simulink model "batteryModelFinal2019a"  (R2019a)
settings: Solver=VariableStepAuto  StartTime=0.0  StopTime=650  RelTol=1e-3
InitFcn:
  | load('batteryModelNew.mat');
  | load('soc_ocv_new.mat');
  | load('currentUAV.mat');
  | 
  | 
  | Q      = battery.QParam; % total capacity in mAh
  | n       = battery.etaParam; % coulombic efficiency
  | M      = battery.MParam; % dynamic hysteresis volts factor
  | Mo     = battery.M0Param; % instant hysteresis volts factor
  | Ro     = battery.R0Param; % internal resistance
  | R       = [battery.RCParam(1)]; % diffusion / warburg impedence, pairs with C
  | C       = [battery.RCParam(2)]; % diffusion / warburg impedence, pairs with R
  | g       = battery.GParam;  % gamma, tunes decay in hysteresis
  | dt      = .01; % delta t
  | eod   = battery.EODParam; % final voltage
  | 
  | if length(R) ~= length(C)
  |     error("R and C must be the same length");
  | end
  | 
  | Arc = zeros(length(R));
  | for i = 1:length(R)
  |     Arc(i,i) = exp(-dt/(R(i)*C(i)));
  | end
  | Brc = zeros(length(R), 1);
  | for i = 1:length(R)
  |     Brc(i,1) = 1 - exp(-dt/(R(i)*C(i)));
  | end
  | k = 1; % timestep
  | Io = .1; % current at time k
  | H(k) = exp(-abs((n(k)*Io(k)*g*dt)/Q));
  | 
  | 
  | %Io = current(1:floor(length(current)/2.5));
  | Io = current;
  | 
  | z = 1.0; % soc
  | Ir = zeros(length(R), 1);
  | h = 0.0;
  | v = ones(length(Io));
  | 
  | 
  | soc = zeros(1, length(Io));
  | v = soc;
values from neighbouring files (symbols this model uses):
  battery =     [batteryModel.mat]
  soc_ocv = [3.01299571991 3.22696254321 3.33372423053 3.41002026482 3.47185878204 3.52366305014 3.56834682613 3.60755277958 3.64212119234 3.67146891607 3.6938685759 3.70622742565 ... (101 elements, 1x101)]    [soc_ocv.mat]
libraries: dspsrcs4 x1
settings Model: Creator=tdarrah  LastModifiedBy=tdarrah
settings DebuggingCC: UnderSpecifiedDimensionMsg=warning

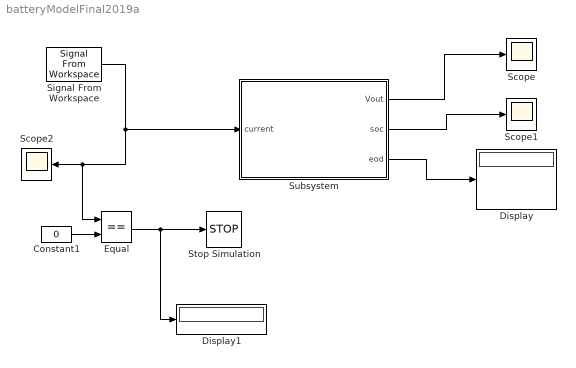
== system batteryModelFinal2019a ==
  Constant1 : Constant  Value=0
  Display : Display
  Display1 : Display
  Equal : RelationalOperator  Operator===  OutDataTypeStr=boolean  RndMeth=Simplest
  Scope : Scope
  Scope1 : Scope
  Scope2 : Scope
  Signal From Workspace : dspsrcs4/Signal From Workspace  X=[Io]  Ts=1/36  nsamps=1  OutputAfterFinalValue=Setting to zero  ignoreOrWarnInputAndFrameLengths=off  OutputFrames=off
  Stop Simulation : Stop
  Subsystem : Subsystem
  wires:
  Signal From Workspace/1 -> Equal/1, Scope2/1, Subsystem/1(current)
  Subsystem/1(Vout) -> Scope/1
  Subsystem/2(soc) -> Scope1/1
  Subsystem/3(eod) -> Display/1
  Constant1/1 -> Equal/2
  Equal/1 -> Display1/1, Stop Simulation/1

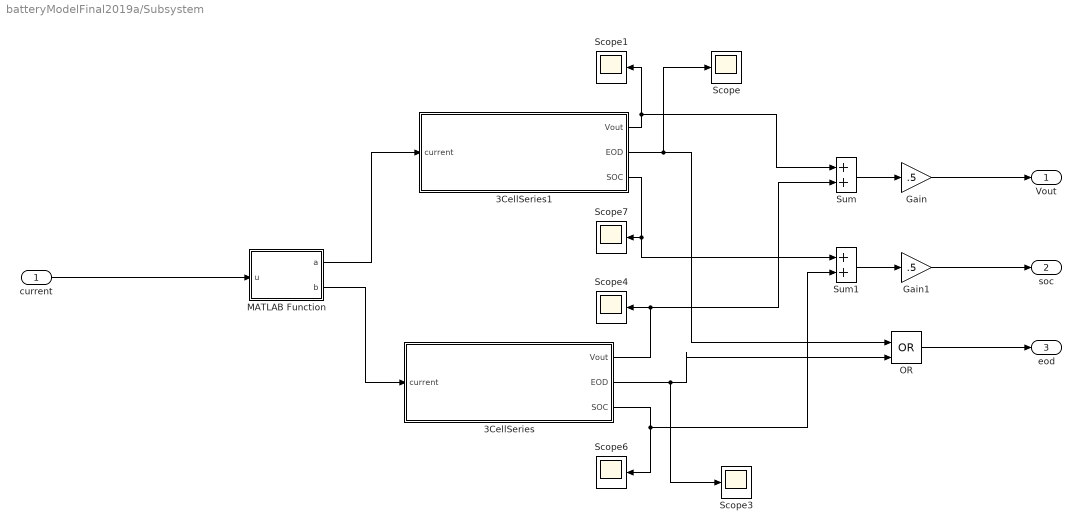
== system batteryModelFinal2019a/Subsystem ==
  current : Inport
  3CellSeries : Subsystem
  3CellSeries1 : Subsystem
  Gain : Gain  Gain=.5
  Gain1 : Gain  Gain=.5
  MATLAB Function : MATLAB Function  TreatAsAtomicUnit=on
  OR : Logic  Operator=OR  IconShape=distinctive  AllPortsSameDT=off  OutDataTypeStr=boolean
  Scope{,1,3..4,6..7} (6 alike) : Scope
  Sum : Sum
  Sum1 : Sum
  Vout : Outport
  soc : Outport  Port=2
  eod : Outport  Port=3
  wires:
  MATLAB Function/2(b) -> 3CellSeries/1(current)
  MATLAB Function/1(a) -> 3CellSeries1/1(current)
  3CellSeries/1(Vout) -> Sum/2, Scope4/1
  Gain/1 -> Vout/1
  3CellSeries1/2(EOD) -> Scope/1, OR/1
  current/1 -> MATLAB Function/1(u)
  3CellSeries1/3(SOC) -> Sum1/1, Scope7/1
  Sum/1 -> Gain/1
  3CellSeries/3(SOC) -> Sum1/2, Scope6/1
  3CellSeries1/1(Vout) -> Sum/1, Scope1/1
  3CellSeries/2(EOD) -> Scope3/1, OR/2
  Sum1/1 -> Gain1/1
  Gain1/1 -> soc/1
  OR/1 -> eod/1

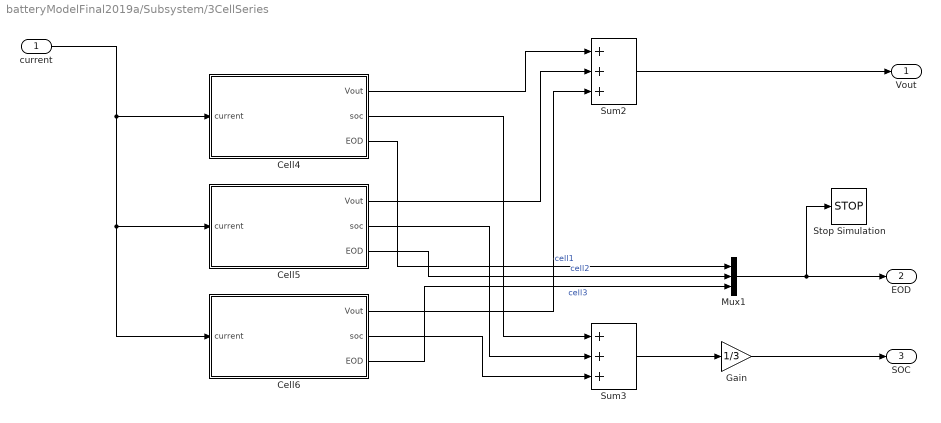
== system batteryModelFinal2019a/Subsystem/3CellSeries ==
  current : Inport
  Cell4 : Subsystem
  Cell5 : Subsystem
  Cell6 : Subsystem
  Gain : Gain  Gain=1/3
  Mux1 : Mux  Inputs=3
  Stop Simulation : Stop
  Sum2 : Sum  Inputs=+++
  Sum3 : Sum  Inputs=+++
  Vout : Outport
  EOD : Outport  Port=2
  SOC : Outport  Port=3
  wires:
  Sum2/1 -> Vout/1
  Cell5/1(Vout) -> Sum2/2
  Cell6/1(Vout) -> Sum2/3
  current/1 -> Cell6/1(current), Cell5/1(current), Cell4/1(current)
  Mux1/1 -> Stop Simulation/1, EOD/1
  Cell4/2(soc) -> Sum3/1
  Cell6/2(soc) -> Sum3/3
  Cell4/1(Vout) -> Sum2/1
  Cell5/2(soc) -> Sum3/2
  Sum3/1 -> Gain/1
  Gain/1 -> SOC/1
  Cell5/3(EOD) -> Mux1/2  "cell2"
  Cell6/3(EOD) -> Mux1/3  "cell3"
  Cell4/3(EOD) -> Mux1/1  "cell1"

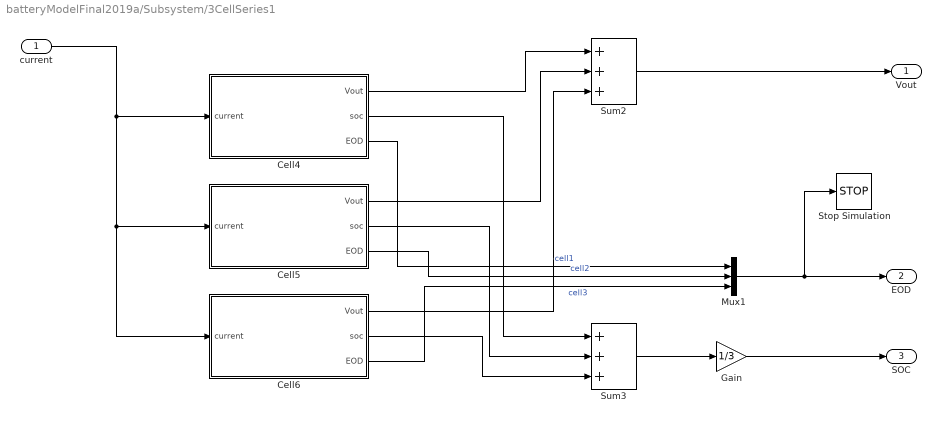
== system batteryModelFinal2019a/Subsystem/3CellSeries1 ==
  current : Inport
  Cell4 : Subsystem
  Cell5 : Subsystem
  Cell6 : Subsystem
  Gain : Gain  Gain=1/3
  Mux1 : Mux  Inputs=3
  Stop Simulation : Stop
  Sum2 : Sum  Inputs=+++
  Sum3 : Sum  Inputs=+++
  Vout : Outport
  EOD : Outport  Port=2
  SOC : Outport  Port=3
  wires:
  Cell6/3(EOD) -> Mux1/3  "cell3"
  Sum2/1 -> Vout/1
  Cell5/1(Vout) -> Sum2/2
  Cell5/3(EOD) -> Mux1/2  "cell2"
  Cell6/1(Vout) -> Sum2/3
  current/1 -> Cell6/1(current), Cell5/1(current), Cell4/1(current)
  Mux1/1 -> Stop Simulation/1, EOD/1
  Cell4/2(soc) -> Sum3/1
  Cell6/2(soc) -> Sum3/3
  Cell4/1(Vout) -> Sum2/1
  Cell5/2(soc) -> Sum3/2
  Sum3/1 -> Gain/1
  Cell4/3(EOD) -> Mux1/1  "cell1"
  Gain/1 -> SOC/1

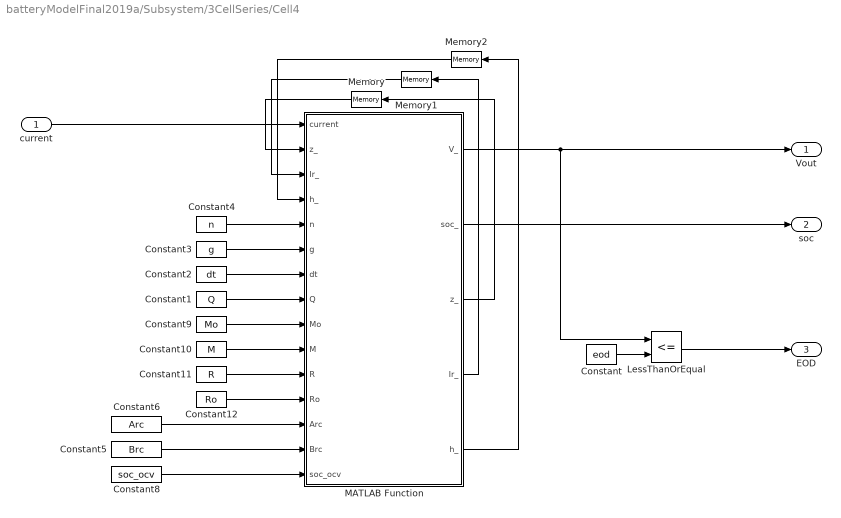
== system batteryModelFinal2019a/Subsystem/3CellSeries/Cell4 ==
  current : Inport
  Constant : Constant  Value=eod
  Constant1 : Constant  Value=Q
  Constant10 : Constant  Value=M
  Constant11 : Constant  Value=R
  Constant12 : Constant  Value=Ro
  Constant2 : Constant  Value=dt
  Constant3 : Constant  Value=g
  Constant4 : Constant  Value=n
  Constant5 : Constant  Value=Brc
  Constant6 : Constant  Value=Arc
  Constant8 : Constant  Value=soc_ocv
  Constant9 : Constant  Value=Mo
  LessThanOrEqual : RelationalOperator  Operator=<=  OutDataTypeStr=boolean  RndMeth=Simplest
  MATLAB Function : MATLAB Function  TreatAsAtomicUnit=on
  Memory : Memory  InitialCondition=1
  Memory1 : Memory
  Memory2 : Memory
  Vout : Outport
  soc : Outport  Port=2
  EOD : Outport  Port=3
  wires:
  MATLAB Function/2(soc_) -> soc/1
  Memory2/1 -> MATLAB Function/4("h_ ")
  Constant11/1 -> MATLAB Function/11(R)
  Constant8/1 -> MATLAB Function/15(soc_ocv)
  Memory/1 -> MATLAB Function/2("z_ ")
  Constant1/1 -> MATLAB Function/8(Q)
  Constant12/1 -> MATLAB Function/12(Ro)
  MATLAB Function/4(Ir_) -> Memory1/1
  Constant5/1 -> MATLAB Function/14(Brc)
  Constant6/1 -> MATLAB Function/13(Arc)
  current/1 -> MATLAB Function/1(current)
  Constant10/1 -> MATLAB Function/10(M)
  Memory1/1 -> MATLAB Function/3("Ir_ ")
  MATLAB Function/3(z_) -> Memory/1
  MATLAB Function/1(V_) -> LessThanOrEqual/1, Vout/1
  MATLAB Function/5(h_) -> Memory2/1
  Constant4/1 -> MATLAB Function/5(n)
  Constant3/1 -> MATLAB Function/6(g)
  Constant9/1 -> MATLAB Function/9(Mo)
  Constant2/1 -> MATLAB Function/7(dt)
  Constant/1 -> LessThanOrEqual/2
  LessThanOrEqual/1 -> EOD/1

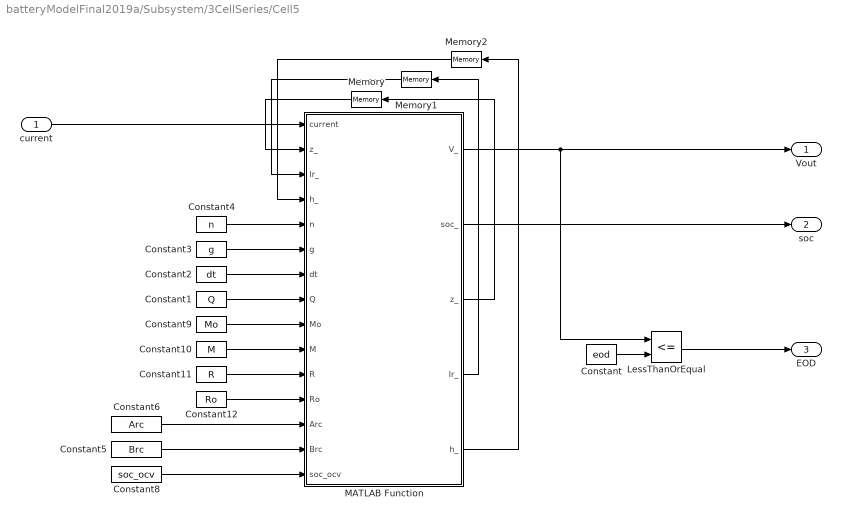
== system batteryModelFinal2019a/Subsystem/3CellSeries/Cell5 ==
  current : Inport
  Constant : Constant  Value=eod
  Constant1 : Constant  Value=Q
  Constant10 : Constant  Value=M
  Constant11 : Constant  Value=R
  Constant12 : Constant  Value=Ro
  Constant2 : Constant  Value=dt
  Constant3 : Constant  Value=g
  Constant4 : Constant  Value=n
  Constant5 : Constant  Value=Brc
  Constant6 : Constant  Value=Arc
  Constant8 : Constant  Value=soc_ocv
  Constant9 : Constant  Value=Mo
  LessThanOrEqual : RelationalOperator  Operator=<=  OutDataTypeStr=boolean  RndMeth=Simplest
  MATLAB Function : MATLAB Function  TreatAsAtomicUnit=on
  Memory : Memory  InitialCondition=1
  Memory1 : Memory
  Memory2 : Memory
  Vout : Outport
  soc : Outport  Port=2
  EOD : Outport  Port=3
  wires:
  MATLAB Function/2(soc_) -> soc/1
  Memory2/1 -> MATLAB Function/4("h_ ")
  Constant11/1 -> MATLAB Function/11(R)
  Constant8/1 -> MATLAB Function/15(soc_ocv)
  Memory/1 -> MATLAB Function/2("z_ ")
  Constant1/1 -> MATLAB Function/8(Q)
  Constant12/1 -> MATLAB Function/12(Ro)
  MATLAB Function/4(Ir_) -> Memory1/1
  Constant5/1 -> MATLAB Function/14(Brc)
  Constant6/1 -> MATLAB Function/13(Arc)
  current/1 -> MATLAB Function/1(current)
  Constant10/1 -> MATLAB Function/10(M)
  Memory1/1 -> MATLAB Function/3("Ir_ ")
  MATLAB Function/3(z_) -> Memory/1
  MATLAB Function/1(V_) -> LessThanOrEqual/1, Vout/1
  MATLAB Function/5(h_) -> Memory2/1
  Constant4/1 -> MATLAB Function/5(n)
  Constant3/1 -> MATLAB Function/6(g)
  Constant9/1 -> MATLAB Function/9(Mo)
  Constant2/1 -> MATLAB Function/7(dt)
  Constant/1 -> LessThanOrEqual/2
  LessThanOrEqual/1 -> EOD/1

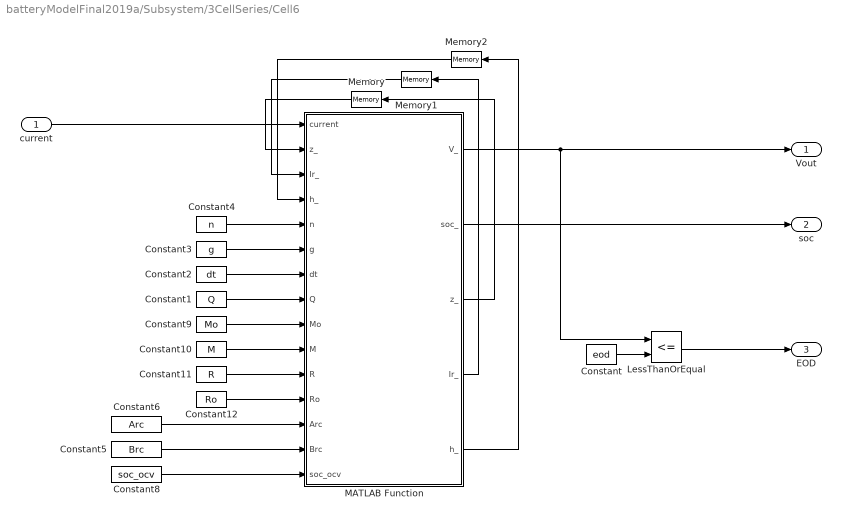
== system batteryModelFinal2019a/Subsystem/3CellSeries/Cell6 ==
  current : Inport
  Constant : Constant  Value=eod
  Constant1 : Constant  Value=Q
  Constant10 : Constant  Value=M
  Constant11 : Constant  Value=R
  Constant12 : Constant  Value=Ro
  Constant2 : Constant  Value=dt
  Constant3 : Constant  Value=g
  Constant4 : Constant  Value=n
  Constant5 : Constant  Value=Brc
  Constant6 : Constant  Value=Arc
  Constant8 : Constant  Value=soc_ocv
  Constant9 : Constant  Value=Mo
  LessThanOrEqual : RelationalOperator  Operator=<=  OutDataTypeStr=boolean  RndMeth=Simplest
  MATLAB Function : MATLAB Function  TreatAsAtomicUnit=on
  Memory : Memory  InitialCondition=1
  Memory1 : Memory
  Memory2 : Memory
  Vout : Outport
  soc : Outport  Port=2
  EOD : Outport  Port=3
  wires:
  MATLAB Function/2(soc_) -> soc/1
  Memory2/1 -> MATLAB Function/4("h_ ")
  Constant11/1 -> MATLAB Function/11(R)
  Constant8/1 -> MATLAB Function/15(soc_ocv)
  Memory/1 -> MATLAB Function/2("z_ ")
  Constant1/1 -> MATLAB Function/8(Q)
  Constant12/1 -> MATLAB Function/12(Ro)
  MATLAB Function/4(Ir_) -> Memory1/1
  Constant5/1 -> MATLAB Function/14(Brc)
  Constant6/1 -> MATLAB Function/13(Arc)
  current/1 -> MATLAB Function/1(current)
  Constant10/1 -> MATLAB Function/10(M)
  Memory1/1 -> MATLAB Function/3("Ir_ ")
  MATLAB Function/3(z_) -> Memory/1
  MATLAB Function/1(V_) -> LessThanOrEqual/1, Vout/1
  MATLAB Function/5(h_) -> Memory2/1
  Constant4/1 -> MATLAB Function/5(n)
  Constant3/1 -> MATLAB Function/6(g)
  Constant9/1 -> MATLAB Function/9(Mo)
  Constant2/1 -> MATLAB Function/7(dt)
  Constant/1 -> LessThanOrEqual/2
  LessThanOrEqual/1 -> EOD/1

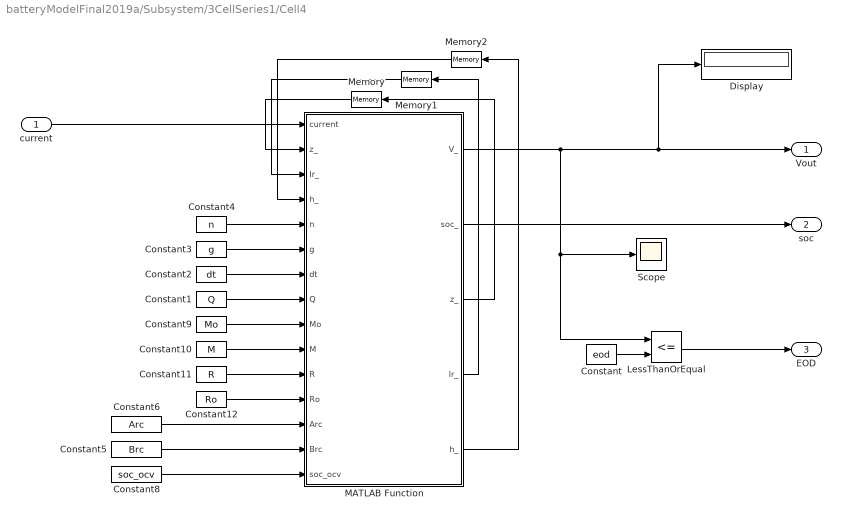
== system batteryModelFinal2019a/Subsystem/3CellSeries1/Cell4 ==
  current : Inport
  Constant : Constant  Value=eod
  Constant1 : Constant  Value=Q
  Constant10 : Constant  Value=M
  Constant11 : Constant  Value=R
  Constant12 : Constant  Value=Ro
  Constant2 : Constant  Value=dt
  Constant3 : Constant  Value=g
  Constant4 : Constant  Value=n
  Constant5 : Constant  Value=Brc
  Constant6 : Constant  Value=Arc
  Constant8 : Constant  Value=soc_ocv
  Constant9 : Constant  Value=Mo
  Display : Display
  LessThanOrEqual : RelationalOperator  Operator=<=  OutDataTypeStr=boolean  RndMeth=Simplest
  MATLAB Function : MATLAB Function  TreatAsAtomicUnit=on
  Memory : Memory  InitialCondition=1
  Memory1 : Memory
  Memory2 : Memory
  Scope : Scope
  Vout : Outport
  soc : Outport  Port=2
  EOD : Outport  Port=3
  wires:
  MATLAB Function/2(soc_) -> soc/1
  Memory2/1 -> MATLAB Function/4("h_ ")
  Constant11/1 -> MATLAB Function/11(R)
  Constant8/1 -> MATLAB Function/15(soc_ocv)
  Memory/1 -> MATLAB Function/2("z_ ")
  Constant1/1 -> MATLAB Function/8(Q)
  Constant12/1 -> MATLAB Function/12(Ro)
  MATLAB Function/4(Ir_) -> Memory1/1
  Constant5/1 -> MATLAB Function/14(Brc)
  Constant6/1 -> MATLAB Function/13(Arc)
  current/1 -> MATLAB Function/1(current)
  Constant10/1 -> MATLAB Function/10(M)
  Memory1/1 -> MATLAB Function/3("Ir_ ")
  MATLAB Function/3(z_) -> Memory/1
  MATLAB Function/1(V_) -> Scope/1, LessThanOrEqual/1, Display/1, Vout/1
  MATLAB Function/5(h_) -> Memory2/1
  Constant4/1 -> MATLAB Function/5(n)
  Constant3/1 -> MATLAB Function/6(g)
  Constant9/1 -> MATLAB Function/9(Mo)
  Constant2/1 -> MATLAB Function/7(dt)
  Constant/1 -> LessThanOrEqual/2
  LessThanOrEqual/1 -> EOD/1

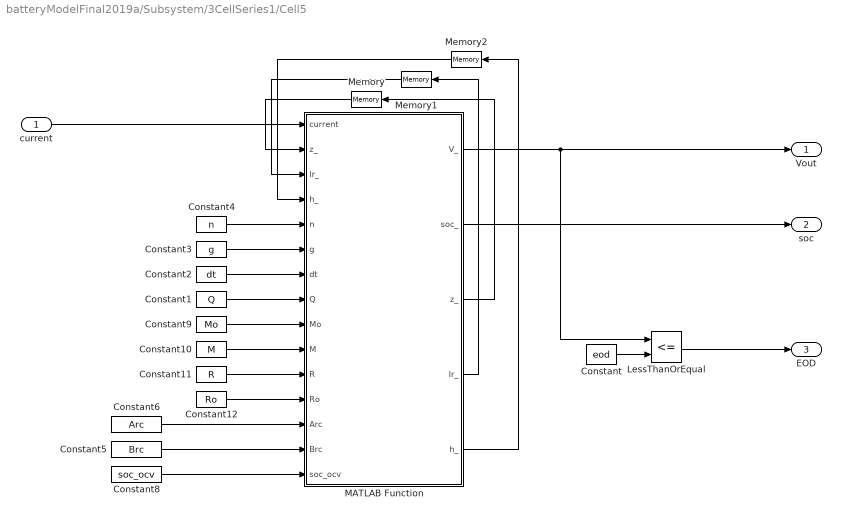
== system batteryModelFinal2019a/Subsystem/3CellSeries1/Cell5 ==
  current : Inport
  Constant : Constant  Value=eod
  Constant1 : Constant  Value=Q
  Constant10 : Constant  Value=M
  Constant11 : Constant  Value=R
  Constant12 : Constant  Value=Ro
  Constant2 : Constant  Value=dt
  Constant3 : Constant  Value=g
  Constant4 : Constant  Value=n
  Constant5 : Constant  Value=Brc
  Constant6 : Constant  Value=Arc
  Constant8 : Constant  Value=soc_ocv
  Constant9 : Constant  Value=Mo
  LessThanOrEqual : RelationalOperator  Operator=<=  OutDataTypeStr=boolean  RndMeth=Simplest
  MATLAB Function : MATLAB Function  TreatAsAtomicUnit=on
  Memory : Memory  InitialCondition=1
  Memory1 : Memory
  Memory2 : Memory
  Vout : Outport
  soc : Outport  Port=2
  EOD : Outport  Port=3
  wires:
  MATLAB Function/2(soc_) -> soc/1
  Memory2/1 -> MATLAB Function/4("h_ ")
  Constant11/1 -> MATLAB Function/11(R)
  Constant8/1 -> MATLAB Function/15(soc_ocv)
  Memory/1 -> MATLAB Function/2("z_ ")
  Constant1/1 -> MATLAB Function/8(Q)
  Constant12/1 -> MATLAB Function/12(Ro)
  MATLAB Function/4(Ir_) -> Memory1/1
  Constant5/1 -> MATLAB Function/14(Brc)
  Constant6/1 -> MATLAB Function/13(Arc)
  current/1 -> MATLAB Function/1(current)
  Constant10/1 -> MATLAB Function/10(M)
  Memory1/1 -> MATLAB Function/3("Ir_ ")
  MATLAB Function/3(z_) -> Memory/1
  MATLAB Function/1(V_) -> LessThanOrEqual/1, Vout/1
  MATLAB Function/5(h_) -> Memory2/1
  Constant4/1 -> MATLAB Function/5(n)
  Constant3/1 -> MATLAB Function/6(g)
  Constant9/1 -> MATLAB Function/9(Mo)
  Constant2/1 -> MATLAB Function/7(dt)
  Constant/1 -> LessThanOrEqual/2
  LessThanOrEqual/1 -> EOD/1

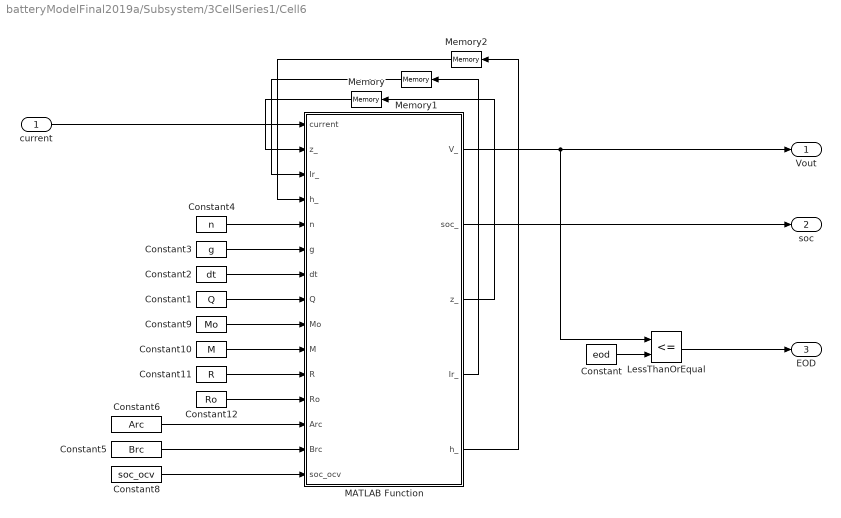
== system batteryModelFinal2019a/Subsystem/3CellSeries1/Cell6 ==
  current : Inport
  Constant : Constant  Value=eod
  Constant1 : Constant  Value=Q
  Constant10 : Constant  Value=M
  Constant11 : Constant  Value=R
  Constant12 : Constant  Value=Ro
  Constant2 : Constant  Value=dt
  Constant3 : Constant  Value=g
  Constant4 : Constant  Value=n
  Constant5 : Constant  Value=Brc
  Constant6 : Constant  Value=Arc
  Constant8 : Constant  Value=soc_ocv
  Constant9 : Constant  Value=Mo
  LessThanOrEqual : RelationalOperator  Operator=<=  OutDataTypeStr=boolean  RndMeth=Simplest
  MATLAB Function : MATLAB Function  TreatAsAtomicUnit=on
  Memory : Memory  InitialCondition=1
  Memory1 : Memory
  Memory2 : Memory
  Vout : Outport
  soc : Outport  Port=2
  EOD : Outport  Port=3
  wires:
  MATLAB Function/2(soc_) -> soc/1
  Memory2/1 -> MATLAB Function/4("h_ ")
  Constant11/1 -> MATLAB Function/11(R)
  Constant8/1 -> MATLAB Function/15(soc_ocv)
  Memory/1 -> MATLAB Function/2("z_ ")
  Constant1/1 -> MATLAB Function/8(Q)
  Constant12/1 -> MATLAB Function/12(Ro)
  MATLAB Function/4(Ir_) -> Memory1/1
  Constant5/1 -> MATLAB Function/14(Brc)
  Constant6/1 -> MATLAB Function/13(Arc)
  current/1 -> MATLAB Function/1(current)
  Constant10/1 -> MATLAB Function/10(M)
  Memory1/1 -> MATLAB Function/3("Ir_ ")
  MATLAB Function/3(z_) -> Memory/1
  MATLAB Function/1(V_) -> LessThanOrEqual/1, Vout/1
  MATLAB Function/5(h_) -> Memory2/1
  Constant4/1 -> MATLAB Function/5(n)
  Constant3/1 -> MATLAB Function/6(g)
  Constant9/1 -> MATLAB Function/9(Mo)
  Constant2/1 -> MATLAB Function/7(dt)
  Constant/1 -> LessThanOrEqual/2
  LessThanOrEqual/1 -> EOD/1

== matlab function batteryModelFinal2019a/Subsystem/3CellSeries1/Cell4/MATLAB Function ==
  data: current input; V_ output; z_ input; Ir_ input; h_ input; soc_ output; z_ output; Ir_ output; h_ output; n input; g input; dt input; Q input; Mo input; M input; R input; Ro input; Arc input; Brc input; soc_ocv input
function [V_, soc_, z_, Ir_, h_]= batterySim(current, z_, Ir_, h_, n, g, dt, Q, Mo, M, R, Ro, Arc, Brc, soc_ocv)
    soc_ = 1.0;
    V_ = 4.2;
    z_dot = z_ - ((n*dt)/Q)*current;
    Ir_dot = Arc*Ir_ + Brc*current;
    H = exp(-abs((n*current*g*dt)/Q));
    h_dot = H*h_ + (H-1)*sign(current);
    z_ = z_dot;
    Ir_ = Ir_dot;
    h_ = h_dot;
    soc_ = (z_ + 31.8816) /(1.0 + 31.8816);
    idx = ceil(soc_*100) +1;
    V_ = (soc_ocv(idx) + Mo*sign(current) + M*h_ - sum(R*Ir_) - Ro*current);

== matlab function batteryModelFinal2019a/Subsystem/3CellSeries1/Cell5/MATLAB Function ==
  data: current input; V_ output; z_ input; Ir_ input; h_ input; soc_ output; z_ output; Ir_ output; h_ output; n input; g input; dt input; Q input; Mo input; M input; R input; Ro input; Arc input; Brc input; soc_ocv input
function [V_, soc_, z_, Ir_, h_]= batterySim(current, z_, Ir_, h_, n, g, dt, Q, Mo, M, R, Ro, Arc, Brc, soc_ocv)
    soc_ = 1.0;
    V_ = 4.2;
    z_dot = z_ - ((n*dt)/Q)*current;
    Ir_dot = Arc*Ir_ + Brc*current;
    H = exp(-abs((n*current*g*dt)/Q));
    h_dot = H*h_ + (H-1)*sign(current);
    z_ = z_dot;
    Ir_ = Ir_dot;
    h_ = h_dot;
    soc_ = (z_ + 31.8816) /(1.0 + 31.8816);
    idx = ceil(soc_*100) +1;
    V_ = (soc_ocv(idx) + Mo*sign(current) + M*h_ - sum(R*Ir_) - Ro*current);

== matlab function batteryModelFinal2019a/Subsystem/3CellSeries1/Cell6/MATLAB Function ==
  data: current input; V_ output; z_ input; Ir_ input; h_ input; soc_ output; z_ output; Ir_ output; h_ output; n input; g input; dt input; Q input; Mo input; M input; R input; Ro input; Arc input; Brc input; soc_ocv input
function [V_, soc_, z_, Ir_, h_]= batterySim(current, z_, Ir_, h_, n, g, dt, Q, Mo, M, R, Ro, Arc, Brc, soc_ocv)
    soc_ = 1.0;
    V_ = 4.2;
    z_dot = z_ - ((n*dt)/Q)*current;
    Ir_dot = Arc*Ir_ + Brc*current;
    H = exp(-abs((n*current*g*dt)/Q));
    h_dot = H*h_ + (H-1)*sign(current);
    z_ = z_dot;
    Ir_ = Ir_dot;
    h_ = h_dot;
    soc_ = (z_ + 31.8816) /(1.0 + 31.8816);
    idx = ceil(soc_*100) +1;
    V_ = (soc_ocv(idx) + Mo*sign(current) + M*h_ - sum(R*Ir_) - Ro*current);

== matlab function batteryModelFinal2019a/Subsystem/3CellSeries/Cell4/MATLAB Function ==
  data: current input; V_ output; z_ input; Ir_ input; h_ input; soc_ output; z_ output; Ir_ output; h_ output; n input; g input; dt input; Q input; Mo input; M input; R input; Ro input; Arc input; Brc input; soc_ocv input
function [V_, soc_, z_, Ir_, h_]= batterySim(current, z_, Ir_, h_, n, g, dt, Q, Mo, M, R, Ro, Arc, Brc, soc_ocv)
    soc_ = 1.0;
    V_ = 4.2;
    z_dot = z_ - ((n*dt)/Q)*current;
    Ir_dot = Arc*Ir_ + Brc*current;
    H = exp(-abs((n*current*g*dt)/Q));
    h_dot = H*h_ + (H-1)*sign(current);
    z_ = z_dot;
    Ir_ = Ir_dot;
    h_ = h_dot;
    soc_ = (z_ + 31.8816) /(1.0 + 31.8816);
    idx = ceil(soc_*100) +1;
    V_ = (soc_ocv(idx) + Mo*sign(current) + M*h_ - sum(R*Ir_) - Ro*current);

== matlab function batteryModelFinal2019a/Subsystem/3CellSeries/Cell5/MATLAB Function ==
  data: current input; V_ output; z_ input; Ir_ input; h_ input; soc_ output; z_ output; Ir_ output; h_ output; n input; g input; dt input; Q input; Mo input; M input; R input; Ro input; Arc input; Brc input; soc_ocv input
function [V_, soc_, z_, Ir_, h_]= batterySim(current, z_, Ir_, h_, n, g, dt, Q, Mo, M, R, Ro, Arc, Brc, soc_ocv)
    soc_ = 1.0;
    V_ = 4.2;
    z_dot = z_ - ((n*dt)/Q)*current;
    Ir_dot = Arc*Ir_ + Brc*current;
    H = exp(-abs((n*current*g*dt)/Q));
    h_dot = H*h_ + (H-1)*sign(current);
    z_ = z_dot;
    Ir_ = Ir_dot;
    h_ = h_dot;
    soc_ = (z_ + 31.8816) /(1.0 + 31.8816);
    idx = ceil(soc_*100) +1;
    V_ = (soc_ocv(idx) + Mo*sign(current) + M*h_ - sum(R*Ir_) - Ro*current);

== matlab function batteryModelFinal2019a/Subsystem/3CellSeries/Cell6/MATLAB Function ==
  data: current input; V_ output; z_ input; Ir_ input; h_ input; soc_ output; z_ output; Ir_ output; h_ output; n input; g input; dt input; Q input; Mo input; M input; R input; Ro input; Arc input; Brc input; soc_ocv input
function [V_, soc_, z_, Ir_, h_]= batterySim(current, z_, Ir_, h_, n, g, dt, Q, Mo, M, R, Ro, Arc, Brc, soc_ocv)
    soc_ = 1.0;
    V_ = 4.2;
    z_dot = z_ - ((n*dt)/Q)*current;
    Ir_dot = Arc*Ir_ + Brc*current;
    H = exp(-abs((n*current*g*dt)/Q));
    h_dot = H*h_ + (H-1)*sign(current);
    z_ = z_dot;
    Ir_ = Ir_dot;
    h_ = h_dot;
    soc_ = (z_ + 31.8816) /(1.0 + 31.8816);
    idx = ceil(soc_*100) +1;
    V_ = (soc_ocv(idx) + Mo*sign(current) + M*h_ - sum(R*Ir_) - Ro*current);

== matlab function batteryModelFinal2019a/Subsystem/MATLAB Function ==
  data: u input; a output; b output
function [a,b]= fcn(u)

a = u/2;
b = u/2;
